simulink model "ManipRoboticoRegolazioneSpazioGiunti_TuningGuadagni"  (R2025b)
settings: Solver=VariableStepAuto  StartTime=0.0  StopTime=10  RelTol=1e-3
settings Model: Creator=arman  LastModifiedBy=Armando

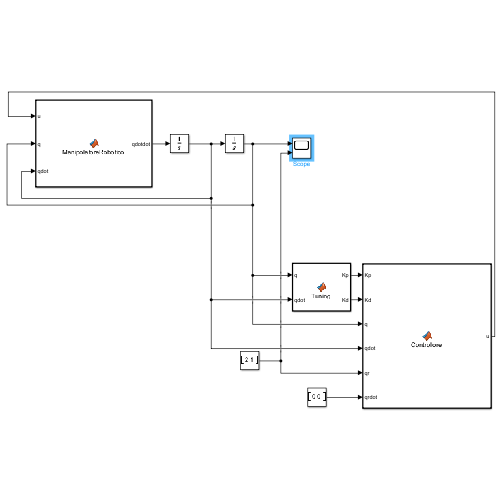
[thumbnail: Simulink's stored preview of the top-level diagram]
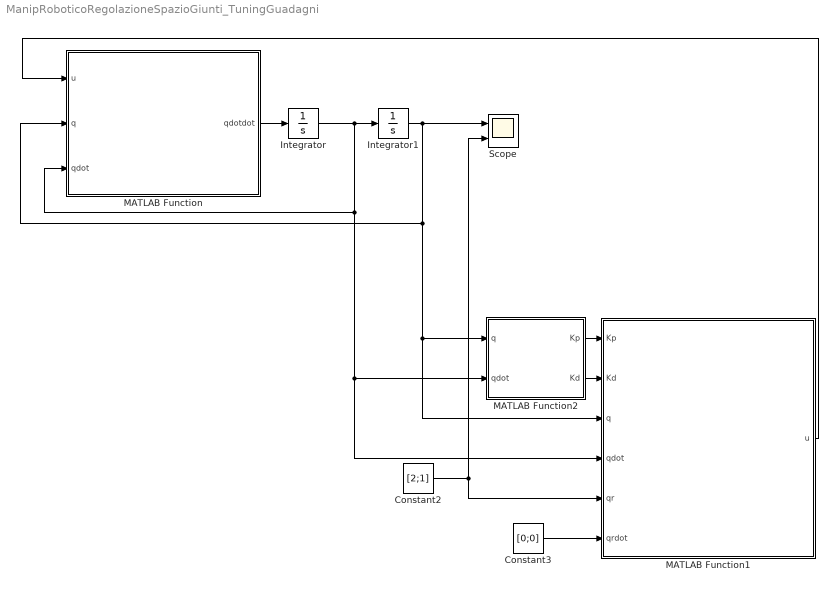
== system ManipRoboticoRegolazioneSpazioGiunti_TuningGuadagni ==
  Constant2 : Constant  Value=[2;1]
  Constant3 : Constant  Value=[0;0]
  Integrator : Integrator  InitialCondition=[0;0]
  Integrator1 : Integrator  InitialCondition=[0;0]
  MATLAB Function : MATLAB Function  TreatAsAtomicUnit=on
  MATLAB Function1 : MATLAB Function  TreatAsAtomicUnit=on
  MATLAB Function2 : MATLAB Function  TreatAsAtomicUnit=on
  Scope : Scope  NumInputPorts=2
      settings: ActiveDisplayYMinimum=-0.95255889776937808  ActiveDisplayYMaximum=3.0170910189312918
  wires:
  MATLAB Function/1(qdotdot) -> Integrator/1
  Integrator/1 -> Integrator1/1, MATLAB Function1/4(qdot), MATLAB Function2/2(qdot), MATLAB Function/3(qdot)
  Integrator1/1 -> Scope/1, MATLAB Function1/3(q), MATLAB Function2/1(q), MATLAB Function/2(q)
  MATLAB Function1/1(u) -> MATLAB Function/1(u)
  Constant2/1 -> Scope/2, MATLAB Function1/5(qr)
  Constant3/1 -> MATLAB Function1/6(qrdot)
  MATLAB Function2/2(Kd) -> MATLAB Function1/2(Kd)
  MATLAB Function2/1(Kp) -> MATLAB Function1/1(Kp)

== matlab function ManipRoboticoRegolazioneSpazioGiunti_TuningGuadagni/MATLAB Function1 ==
  data: Kp input; Kd input; u output; q input; qdot input; qr input; qrdot input
function u = Controllore(Kp,Kd,q,qdot,qr,qrdot)
e = q - qr;
edot = qdot - qrdot;
[B, C, g, F] = calculateMatrixRobotRR(q,qdot);
u =g  - Kp.*e - Kd.*edot;

== matlab function ManipRoboticoRegolazioneSpazioGiunti_TuningGuadagni/MATLAB Function ==
  data: u input; q input; qdotdot output; qdot input
function qdotdot = ManipolatoreRobotico(u,q,qdot)
[B, C, g, F] = calculateMatrixRobotRR(q,qdot);
qdotdot = B \ (u - (C * qdot) - g - F);

== matlab function ManipRoboticoRegolazioneSpazioGiunti_TuningGuadagni/MATLAB Function2 ==
  data: q input; Kp output; qdot input; Kd output
function [Kp,Kd] = Tuning(q,qdot)
[B, C, g, F] = calculateMatrixRobotRR(q,qdot);
xi =0.7;
Ts=3;
wn = 4/(xi * Ts);

B_giunti = [B(1,1);B(2,2)];
Kd = 2 * B_giunti * xi * wn;
Kp = B_giunti * (wn)^2;
